simulink model "road_wheel_and_actuator_dynamics"  (R2022b)
settings: Solver=VariableStepAuto  StartTime=0.0  StopTime=10.0  RelTol=1e-3
undefined symbols (not defined in the file): Bm2, Br, Btr, G, Im2, Jtr, Ke2, kp, kr, ks, Kt2, ktr, L2, Mr, N, n, n1, R2, rp, to
libraries: simulink_extras x1
settings Model: Creator=Timothy  LastModifiedBy=Timothy

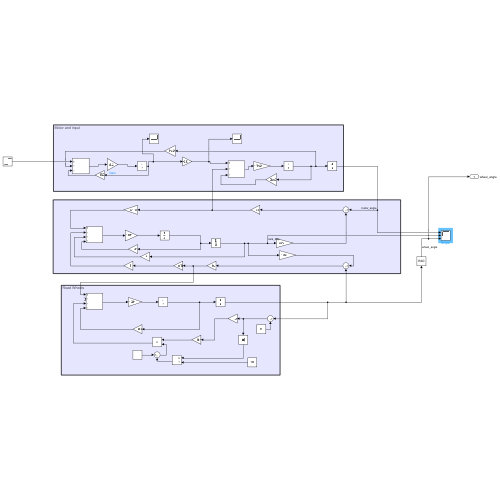
[thumbnail: Simulink's stored preview of the top-level diagram]
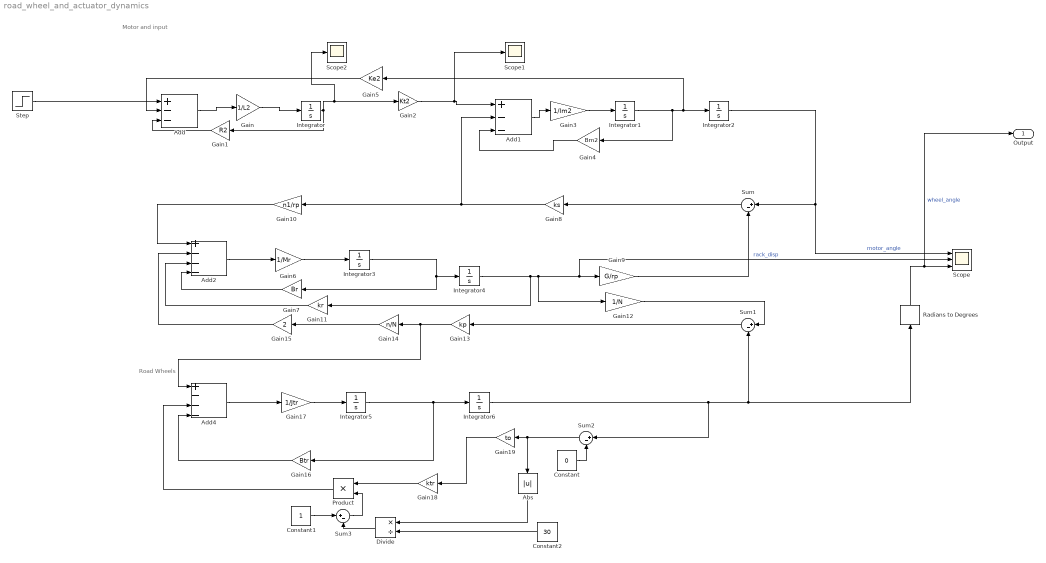
== system road_wheel_and_actuator_dynamics ==
  note: Road Wheels
  note: Motor and input
  Abs : Abs  SaturateOnIntegerOverflow=off
  Add : Sum  Inputs=+--
  Add1 : Sum  Inputs=+--
  Add2 : Sum  Inputs=+---
  Add4 : Sum  Inputs=+---
  Constant : Constant  Value=0
  Constant1 : Constant
  Constant2 : Constant  Value=30
  Divide : Product  Inputs=*/
  Gain : Gain  Gain=1/L2
  Gain1 : Gain  Gain=R2
  Gain10 : Gain  Gain=n1/rp
  Gain11 : Gain  Gain=kr
  Gain12 : Gain  Gain=1/N
  Gain13 : Gain  Gain=kp
  Gain14 : Gain  Gain=n/N
  Gain15 : Gain  Gain=2
  Gain16 : Gain  Gain=Btr
  Gain17 : Gain  Gain=1/Jtr
  Gain18 : Gain  Gain=ktr
  Gain19 : Gain  Gain=to
  Gain2 : Gain  Gain=Kt2
  Gain3 : Gain  Gain=1/Im2
  Gain4 : Gain  Gain=Bm2
  Gain5 : Gain  Gain=Ke2
  Gain6 : Gain  Gain=1/Mr
  Gain7 : Gain  Gain=Br
  Gain8 : Gain  Gain=ks
  Gain9 : Gain  Gain=G/rp
  Integrator{,1..6} (7 alike) : Integrator
  Product : Product
  Radians to Degrees : simulink_extras/Transformations/Radians to Degrees
  Scope : Scope  NumInputPorts=3
  Scope1 : Scope
  Scope2 : Scope
  Step : Step  SampleTime=0
  Sum{,1..3} (4 alike) : Sum  Inputs=|+-
  Output : Outport  SignalName=wheel_angle
  wires:
  Radians to Degrees/1 -> Output/1, Scope/3  "wheel_angle"
  Gain5/1 -> Add/2
  Integrator4/1 -> Gain11/1, Gain12/1, Scope/2, Gain9/1  "rack_disp"
  Abs/1 -> Divide/1
  Step/1 -> Add/1
  Gain4/1 -> Add1/3
  Sum3/1 -> Product/2
  Gain17/1 -> Integrator5/1
  Gain1/1 -> Add/3
  Gain19/1 -> Gain18/1
  Constant1/1 -> Sum3/1
  Divide/1 -> Sum3/2
  Integrator6/1 -> Radians to Degrees/1, Sum1/2, Sum2/1
  Gain18/1 -> Product/1
  Integrator3/1 -> Gain7/1, Integrator4/1
  Gain16/1 -> Add4/4
  Add2/1 -> Gain6/1
  Gain9/1 -> Sum/2
  Sum/1 -> Gain8/1
  Gain14/1 -> Gain15/1
  Gain8/1 -> Gain10/1, Add1/2
  Sum1/1 -> Gain13/1
  Gain13/1 -> Add4/1, Gain14/1
  Gain10/1 -> Add2/1
  Sum2/1 -> Abs/1, Gain19/1
  Constant/1 -> Sum2/2
  Gain7/1 -> Add2/4
  Constant2/1 -> Divide/2
  Integrator5/1 -> Gain16/1, Integrator6/1
  Add/1 -> Gain/1
  Integrator/1 -> Gain1/1, Gain2/1, Scope2/1
  Product/1 -> Add4/3
  Gain2/1 -> Scope1/1, Add1/1
  Gain15/1 -> Add2/2
  Integrator2/1 -> Sum/1, Scope/1  "motor_angle"
  Gain6/1 -> Integrator3/1
  Add4/1 -> Gain17/1
  Add1/1 -> Gain3/1
  Gain12/1 -> Sum1/1
  Gain/1 -> Integrator/1
  Gain3/1 -> Integrator1/1
  Gain11/1 -> Add2/3
  Integrator1/1 -> Gain4/1, Gain5/1, Integrator2/1
